simulink subsystem "sim_battery_subsystem"  (R2023a)
settings: Solver=VariableStepAuto  StartTime=0.0  StopTime=10.0  RelTol=1e-3
undefined symbols (not defined in the file or in its folder): battery_builder_rtmsupport, gcbh
libraries: nesl_utility x14, GD_Batterymodel_6_lib x8, fl_lib x7, BatteryCurrentManagement x1, batt_lib x1, BatteryBalancing x1, simulink x1, SimscapeFluids_lib x1
(part 2 of 2)

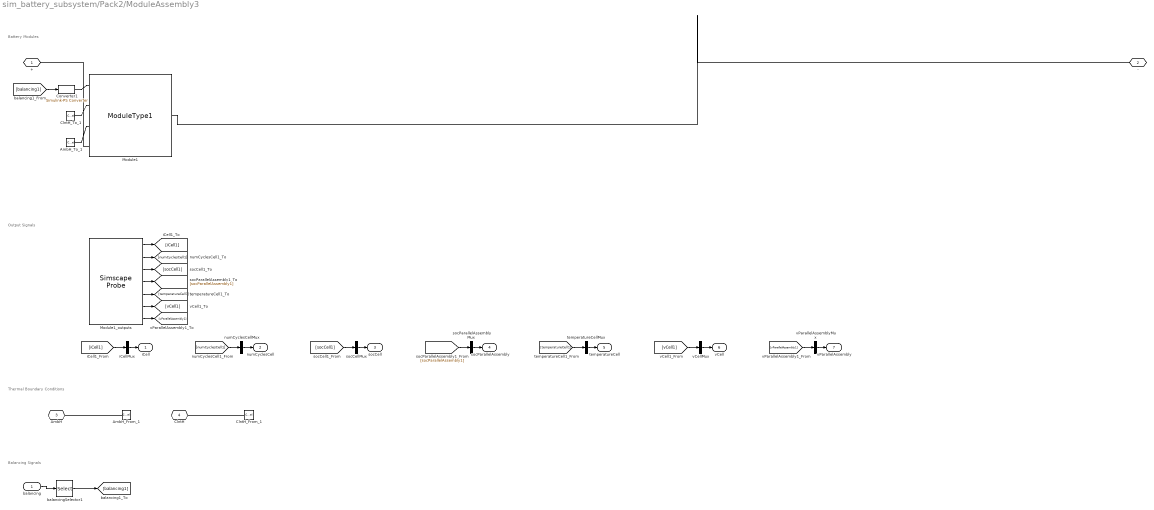
== system sim_battery_subsystem/Pack2/ModuleAssembly3 ==
  note: Balancing Signals
  note: Thermal Boundary Conditions
  note: Output Signals
  note: Battery Modules
  balancing : Inport  PortDimensions=14
  AmbH_From_1 : ConnectionLabel  Label=ambH_1
  AmbH_To_1 : ConnectionLabel  Label=ambH_1
  ClntH_From_1 : ConnectionLabel  Label=clntH_1
  ClntH_To_1 : ConnectionLabel  Label=clntH_1
  Converter1 : nesl_utility/Simulink-PS Converter  PhysicalDomain=network_engine_domain  SubClassName=ps_input  LeftPortType=input  RightPortType=output  PseudoPeriodic=off  Frequencies=[]  NoiseDistribution=none  NoiseParameters=[]  Unit=1  AffineConversion=off  FilteringAndDerivatives=provide  SimscapeFilterOrder=1  InputFilterTimeConstant=0.001  UdotUserProvided=0
  Module1 : GD_Batterymodel_6_lib/Modules/ModuleType1  SOC_vecCell=ModuleType1.SOC_vecCell  T_vecCell=ModuleType1.T_vecCell K  V0_matCell=ModuleType1.V0_matCell V  V_rangeCell=ModuleType1.V_rangeCell V  R0_matCell=ModuleType1.R0_matCell Ohm  AHCell=ModuleType1.AHCell A*hr  extrapolation_optionCell=simscape.enum.extrapolation.nearest  R1_matCell=ModuleType1.R1_matCell Ohm  tau1_matCell=ModuleType1.tau1_matCell s  R2_matCell=ModuleType1.R2_matCell Ohm  tau2_matCell=ModuleType1.tau2_matCell s  thermal_massCell=ModuleType1.thermal_massCell J/K  CoolantResistance=ModuleType1.CoolantResistance K/W  AmbientResistance=ModuleType1.AmbientResistance K/W  CellBalancingClosedResistance=ModuleType1.CellBalancingClosedResistance Ohm  CellBalancingOpenConductance=ModuleType1.CellBalancingOpenConductance 1/Ohm  CellBalancingThreshold=ModuleType1.CellBalancingThreshold  CellBalancingResistance=ModuleType1.CellBalancingResistance Ohm  P=3  S=14  iCell_specify=on  iCell_priority=None  iCell=ModuleAssembly3.Module1.iCell A  iCell_nominal_specify=off  iCell_nominal_unit=A  iCell_nominal_value=1  vCell_specify=on  vCell_priority=None  vCell=ModuleAssembly3.Module1.vCell V  vCell_nominal_specify=off  vCell_nominal_unit=V  vCell_nominal_value=1  socCell_specify=on  socCell_priority=High  socCell=ModuleAssembly3.Module1.socCell  socCell_nominal_specify=off  socCell_nominal_unit=1  socCell_nominal_value=1  numCyclesCell_specify=on  numCyclesCell_priority=High  numCyclesCell=ModuleAssembly3.Module1.numCyclesCell  numCyclesCell_nominal_specify=off  numCyclesCell_nominal_unit=1  numCyclesCell_nominal_value=1  temperatureCell_specify=on  temperatureCell_priority=High  temperatureCell=ModuleAssembly3.Module1.temperatureCell K  temperatureCell_nominal_specify=off  temperatureCell_nominal_unit=K  temperatureCell_nominal_value=1  vParallelAssembly_specify=on  vParallelAssembly_priority=None  vParallelAssembly=ModuleAssembly3.Module1.vParallelAssembly V  vParallelAssembly_nominal_specify=off  vParallelAssembly_nominal_unit=V  vParallelAssembly_nominal_value=1  socParallelAssembly_specify=on  socParallelAssembly_priority=None  socParallelAssembly=ModuleAssembly3.Module1.socParallelAssembly  socParallelAssembly_nominal_specify=off  socParallelAssembly_nominal_unit=1  socParallelAssembly_nominal_value=1
      settings: InternalSimscapePortConfiguration="{\"Bottom\":[{\"id\":\"n\",\"label\":\"-\",\"type\":\"foundation.electrical.electrical\"}],\"Left\":[{\"id\":\"enableCellBalancing\",\"label\":\"CB\",\"type\":\"input\"},{\"id\":\"ClntH\",\"label\":\"CH\",\"type\":\"foundation.thermal.thermal\"},{\"id\":\"AmbH\",\"label\":\"AH\",\"type\":\"foundation.thermal.thermal\"}],\"Right\":[],\"Top\":[{\"id\":\"p\",\"label\":\"+\",\"type\":\"foundation.electrical.electrical\"}]}"
  Module1_outputs : SimscapeProbe  BoundBlock=152  Variables={iCell, numCyclesCell, socCell, socParallelAssembly, temperatureCell, vCell, vParallelAssembly}
  balancingSelector1 : Selector  InputPortWidth=14  IndexOptions=Index vector (dialog)  Indices="[1   2   3   4   5   6   7   8   9  10  11  12  13  14]"  OutputSizes=1
  iCellMux : Mux  Inputs=1
  numCyclesCellMux : Mux  Inputs=1
  socCellMux : Mux  Inputs=1
  socParallelAssemblyMux : Mux  Inputs=1
  temperatureCellMux : Mux  Inputs=1
  vCellMux : Mux  Inputs=1
  vParallelAssemblyMux : Mux  Inputs=1
  + : PMIOPort  Side=Left
  - : PMIOPort  Port=2  Side=Right
  AmbH : PMIOPort  Port=3  Side=Right  ConnectionType=Connection: foundation.thermal.thermal
  ClntH : PMIOPort  Port=4  Side=Right  ConnectionType=Connection: foundation.thermal.thermal
  iCell : Outport
  numCyclesCell : Outport  Port=2
  socCell : Outport  Port=3
  socParallelAssembly : Outport  Port=4
  temperatureCell : Outport  Port=5
  vCell : Outport  Port=6
  vParallelAssembly : Outport  Port=7
  wires:
  balancingSelector1/1 -> [balancing1]
  balancing/1 -> balancingSelector1/1
  [balancing1] -> Converter1/1
  [vParallelAssembly1] -> vParallelAssemblyMux/1
  vParallelAssemblyMux/1 -> vParallelAssembly/1
  Module1_outputs/7 -> [vParallelAssembly1]
  [vCell1] -> vCellMux/1
  vCellMux/1 -> vCell/1
  Module1_outputs/6 -> [vCell1]
  [temperatureCell1] -> temperatureCellMux/1
  temperatureCellMux/1 -> temperatureCell/1
  Module1_outputs/5 -> [temperatureCell1]
  [socParallelAssembly1] -> socParallelAssemblyMux/1
  socParallelAssemblyMux/1 -> socParallelAssembly/1
  Module1_outputs/4 -> [socParallelAssembly1]
  [socCell1] -> socCellMux/1
  socCellMux/1 -> socCell/1
  Module1_outputs/3 -> [socCell1]
  [numCyclesCell1] -> numCyclesCellMux/1
  numCyclesCellMux/1 -> numCyclesCell/1
  Module1_outputs/2 -> [numCyclesCell1]
  [iCell1] -> iCellMux/1
  iCellMux/1 -> iCell/1
  Module1_outputs/1 -> [iCell1]
  connections:
  Converter1/RConn1 -- Module1/LConn1
  ClntH_From_1/LConn1 -- ClntH/RConn1
  ClntH_To_1/LConn1 -- Module1/LConn2
  AmbH_From_1/LConn1 -- AmbH/RConn1
  AmbH_To_1/LConn1 -- Module1/LConn3
  Module1/RConn1 -- -/RConn1
  Module1/LConn4 -- +/RConn1

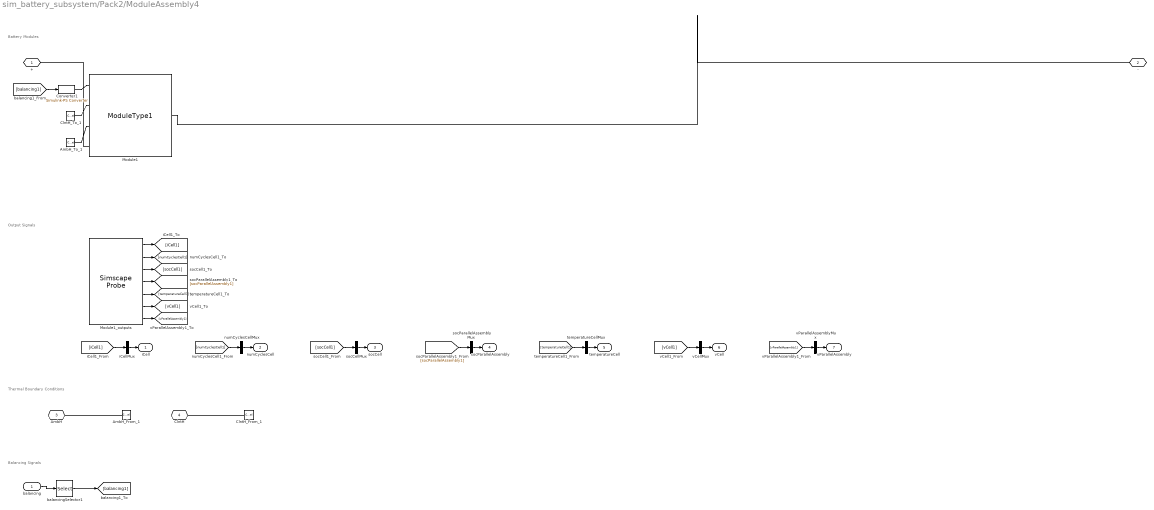
== system sim_battery_subsystem/Pack2/ModuleAssembly4 ==
  note: Balancing Signals
  note: Thermal Boundary Conditions
  note: Output Signals
  note: Battery Modules
  balancing : Inport  PortDimensions=14
  AmbH_From_1 : ConnectionLabel  Label=ambH_1
  AmbH_To_1 : ConnectionLabel  Label=ambH_1
  ClntH_From_1 : ConnectionLabel  Label=clntH_1
  ClntH_To_1 : ConnectionLabel  Label=clntH_1
  Converter1 : nesl_utility/Simulink-PS Converter  PhysicalDomain=network_engine_domain  SubClassName=ps_input  LeftPortType=input  RightPortType=output  PseudoPeriodic=off  Frequencies=[]  NoiseDistribution=none  NoiseParameters=[]  Unit=1  AffineConversion=off  FilteringAndDerivatives=provide  SimscapeFilterOrder=1  InputFilterTimeConstant=0.001  UdotUserProvided=0
  Module1 : GD_Batterymodel_6_lib/Modules/ModuleType1  SOC_vecCell=ModuleType1.SOC_vecCell  T_vecCell=ModuleType1.T_vecCell K  V0_matCell=ModuleType1.V0_matCell V  V_rangeCell=ModuleType1.V_rangeCell V  R0_matCell=ModuleType1.R0_matCell Ohm  AHCell=ModuleType1.AHCell A*hr  extrapolation_optionCell=simscape.enum.extrapolation.nearest  R1_matCell=ModuleType1.R1_matCell Ohm  tau1_matCell=ModuleType1.tau1_matCell s  R2_matCell=ModuleType1.R2_matCell Ohm  tau2_matCell=ModuleType1.tau2_matCell s  thermal_massCell=ModuleType1.thermal_massCell J/K  CoolantResistance=ModuleType1.CoolantResistance K/W  AmbientResistance=ModuleType1.AmbientResistance K/W  CellBalancingClosedResistance=ModuleType1.CellBalancingClosedResistance Ohm  CellBalancingOpenConductance=ModuleType1.CellBalancingOpenConductance 1/Ohm  CellBalancingThreshold=ModuleType1.CellBalancingThreshold  CellBalancingResistance=ModuleType1.CellBalancingResistance Ohm  P=3  S=14  iCell_specify=on  iCell_priority=None  iCell=ModuleAssembly4.Module1.iCell A  iCell_nominal_specify=off  iCell_nominal_unit=A  iCell_nominal_value=1  vCell_specify=on  vCell_priority=None  vCell=ModuleAssembly4.Module1.vCell V  vCell_nominal_specify=off  vCell_nominal_unit=V  vCell_nominal_value=1  socCell_specify=on  socCell_priority=High  socCell=ModuleAssembly4.Module1.socCell  socCell_nominal_specify=off  socCell_nominal_unit=1  socCell_nominal_value=1  numCyclesCell_specify=on  numCyclesCell_priority=High  numCyclesCell=ModuleAssembly4.Module1.numCyclesCell  numCyclesCell_nominal_specify=off  numCyclesCell_nominal_unit=1  numCyclesCell_nominal_value=1  temperatureCell_specify=on  temperatureCell_priority=High  temperatureCell=ModuleAssembly4.Module1.temperatureCell K  temperatureCell_nominal_specify=off  temperatureCell_nominal_unit=K  temperatureCell_nominal_value=1  vParallelAssembly_specify=on  vParallelAssembly_priority=None  vParallelAssembly=ModuleAssembly4.Module1.vParallelAssembly V  vParallelAssembly_nominal_specify=off  vParallelAssembly_nominal_unit=V  vParallelAssembly_nominal_value=1  socParallelAssembly_specify=on  socParallelAssembly_priority=None  socParallelAssembly=ModuleAssembly4.Module1.socParallelAssembly  socParallelAssembly_nominal_specify=off  socParallelAssembly_nominal_unit=1  socParallelAssembly_nominal_value=1
      settings: InternalSimscapePortConfiguration="{\"Bottom\":[{\"id\":\"n\",\"label\":\"-\",\"type\":\"foundation.electrical.electrical\"}],\"Left\":[{\"id\":\"enableCellBalancing\",\"label\":\"CB\",\"type\":\"input\"},{\"id\":\"ClntH\",\"label\":\"CH\",\"type\":\"foundation.thermal.thermal\"},{\"id\":\"AmbH\",\"label\":\"AH\",\"type\":\"foundation.thermal.thermal\"}],\"Right\":[],\"Top\":[{\"id\":\"p\",\"label\":\"+\",\"type\":\"foundation.electrical.electrical\"}]}"
  Module1_outputs : SimscapeProbe  BoundBlock=200  Variables={iCell, numCyclesCell, socCell, socParallelAssembly, temperatureCell, vCell, vParallelAssembly}
  balancingSelector1 : Selector  InputPortWidth=14  IndexOptions=Index vector (dialog)  Indices="[1   2   3   4   5   6   7   8   9  10  11  12  13  14]"  OutputSizes=1
  iCellMux : Mux  Inputs=1
  numCyclesCellMux : Mux  Inputs=1
  socCellMux : Mux  Inputs=1
  socParallelAssemblyMux : Mux  Inputs=1
  temperatureCellMux : Mux  Inputs=1
  vCellMux : Mux  Inputs=1
  vParallelAssemblyMux : Mux  Inputs=1
  + : PMIOPort  Side=Left
  - : PMIOPort  Port=2  Side=Right
  AmbH : PMIOPort  Port=3  Side=Right  ConnectionType=Connection: foundation.thermal.thermal
  ClntH : PMIOPort  Port=4  Side=Right  ConnectionType=Connection: foundation.thermal.thermal
  iCell : Outport
  numCyclesCell : Outport  Port=2
  socCell : Outport  Port=3
  socParallelAssembly : Outport  Port=4
  temperatureCell : Outport  Port=5
  vCell : Outport  Port=6
  vParallelAssembly : Outport  Port=7
  wires:
  balancingSelector1/1 -> [balancing1]
  balancing/1 -> balancingSelector1/1
  [balancing1] -> Converter1/1
  [vParallelAssembly1] -> vParallelAssemblyMux/1
  vParallelAssemblyMux/1 -> vParallelAssembly/1
  Module1_outputs/7 -> [vParallelAssembly1]
  [vCell1] -> vCellMux/1
  vCellMux/1 -> vCell/1
  Module1_outputs/6 -> [vCell1]
  [temperatureCell1] -> temperatureCellMux/1
  temperatureCellMux/1 -> temperatureCell/1
  Module1_outputs/5 -> [temperatureCell1]
  [socParallelAssembly1] -> socParallelAssemblyMux/1
  socParallelAssemblyMux/1 -> socParallelAssembly/1
  Module1_outputs/4 -> [socParallelAssembly1]
  [socCell1] -> socCellMux/1
  socCellMux/1 -> socCell/1
  Module1_outputs/3 -> [socCell1]
  [numCyclesCell1] -> numCyclesCellMux/1
  numCyclesCellMux/1 -> numCyclesCell/1
  Module1_outputs/2 -> [numCyclesCell1]
  [iCell1] -> iCellMux/1
  iCellMux/1 -> iCell/1
  Module1_outputs/1 -> [iCell1]
  connections:
  Converter1/RConn1 -- Module1/LConn1
  ClntH_From_1/LConn1 -- ClntH/RConn1
  ClntH_To_1/LConn1 -- Module1/LConn2
  AmbH_From_1/LConn1 -- AmbH/RConn1
  AmbH_To_1/LConn1 -- Module1/LConn3
  Module1/RConn1 -- -/RConn1
  Module1/LConn4 -- +/RConn1

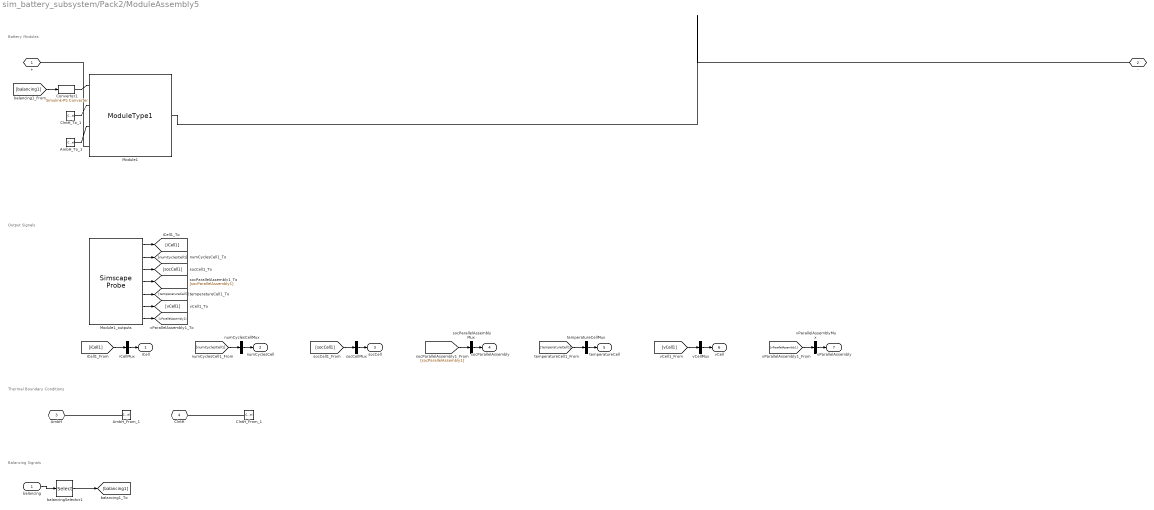
== system sim_battery_subsystem/Pack2/ModuleAssembly5 ==
  note: Balancing Signals
  note: Thermal Boundary Conditions
  note: Output Signals
  note: Battery Modules
  balancing : Inport  PortDimensions=14
  AmbH_From_1 : ConnectionLabel  Label=ambH_1
  AmbH_To_1 : ConnectionLabel  Label=ambH_1
  ClntH_From_1 : ConnectionLabel  Label=clntH_1
  ClntH_To_1 : ConnectionLabel  Label=clntH_1
  Converter1 : nesl_utility/Simulink-PS Converter  PhysicalDomain=network_engine_domain  SubClassName=ps_input  LeftPortType=input  RightPortType=output  PseudoPeriodic=off  Frequencies=[]  NoiseDistribution=none  NoiseParameters=[]  Unit=1  AffineConversion=off  FilteringAndDerivatives=provide  SimscapeFilterOrder=1  InputFilterTimeConstant=0.001  UdotUserProvided=0
  Module1 : GD_Batterymodel_6_lib/Modules/ModuleType1  SOC_vecCell=ModuleType1.SOC_vecCell  T_vecCell=ModuleType1.T_vecCell K  V0_matCell=ModuleType1.V0_matCell V  V_rangeCell=ModuleType1.V_rangeCell V  R0_matCell=ModuleType1.R0_matCell Ohm  AHCell=ModuleType1.AHCell A*hr  extrapolation_optionCell=simscape.enum.extrapolation.nearest  R1_matCell=ModuleType1.R1_matCell Ohm  tau1_matCell=ModuleType1.tau1_matCell s  R2_matCell=ModuleType1.R2_matCell Ohm  tau2_matCell=ModuleType1.tau2_matCell s  thermal_massCell=ModuleType1.thermal_massCell J/K  CoolantResistance=ModuleType1.CoolantResistance K/W  AmbientResistance=ModuleType1.AmbientResistance K/W  CellBalancingClosedResistance=ModuleType1.CellBalancingClosedResistance Ohm  CellBalancingOpenConductance=ModuleType1.CellBalancingOpenConductance 1/Ohm  CellBalancingThreshold=ModuleType1.CellBalancingThreshold  CellBalancingResistance=ModuleType1.CellBalancingResistance Ohm  P=3  S=14  iCell_specify=on  iCell_priority=None  iCell=ModuleAssembly5.Module1.iCell A  iCell_nominal_specify=off  iCell_nominal_unit=A  iCell_nominal_value=1  vCell_specify=on  vCell_priority=None  vCell=ModuleAssembly5.Module1.vCell V  vCell_nominal_specify=off  vCell_nominal_unit=V  vCell_nominal_value=1  socCell_specify=on  socCell_priority=High  socCell=ModuleAssembly5.Module1.socCell  socCell_nominal_specify=off  socCell_nominal_unit=1  socCell_nominal_value=1  numCyclesCell_specify=on  numCyclesCell_priority=High  numCyclesCell=ModuleAssembly5.Module1.numCyclesCell  numCyclesCell_nominal_specify=off  numCyclesCell_nominal_unit=1  numCyclesCell_nominal_value=1  temperatureCell_specify=on  temperatureCell_priority=High  temperatureCell=ModuleAssembly5.Module1.temperatureCell K  temperatureCell_nominal_specify=off  temperatureCell_nominal_unit=K  temperatureCell_nominal_value=1  vParallelAssembly_specify=on  vParallelAssembly_priority=None  vParallelAssembly=ModuleAssembly5.Module1.vParallelAssembly V  vParallelAssembly_nominal_specify=off  vParallelAssembly_nominal_unit=V  vParallelAssembly_nominal_value=1  socParallelAssembly_specify=on  socParallelAssembly_priority=None  socParallelAssembly=ModuleAssembly5.Module1.socParallelAssembly  socParallelAssembly_nominal_specify=off  socParallelAssembly_nominal_unit=1  socParallelAssembly_nominal_value=1
      settings: InternalSimscapePortConfiguration="{\"Bottom\":[{\"id\":\"n\",\"label\":\"-\",\"type\":\"foundation.electrical.electrical\"}],\"Left\":[{\"id\":\"enableCellBalancing\",\"label\":\"CB\",\"type\":\"input\"},{\"id\":\"ClntH\",\"label\":\"CH\",\"type\":\"foundation.thermal.thermal\"},{\"id\":\"AmbH\",\"label\":\"AH\",\"type\":\"foundation.thermal.thermal\"}],\"Right\":[],\"Top\":[{\"id\":\"p\",\"label\":\"+\",\"type\":\"foundation.electrical.electrical\"}]}"
  Module1_outputs : SimscapeProbe  BoundBlock=248  Variables={iCell, numCyclesCell, socCell, socParallelAssembly, temperatureCell, vCell, vParallelAssembly}
  balancingSelector1 : Selector  InputPortWidth=14  IndexOptions=Index vector (dialog)  Indices="[1   2   3   4   5   6   7   8   9  10  11  12  13  14]"  OutputSizes=1
  iCellMux : Mux  Inputs=1
  numCyclesCellMux : Mux  Inputs=1
  socCellMux : Mux  Inputs=1
  socParallelAssemblyMux : Mux  Inputs=1
  temperatureCellMux : Mux  Inputs=1
  vCellMux : Mux  Inputs=1
  vParallelAssemblyMux : Mux  Inputs=1
  + : PMIOPort  Side=Left
  - : PMIOPort  Port=2  Side=Right
  AmbH : PMIOPort  Port=3  Side=Right  ConnectionType=Connection: foundation.thermal.thermal
  ClntH : PMIOPort  Port=4  Side=Right  ConnectionType=Connection: foundation.thermal.thermal
  iCell : Outport
  numCyclesCell : Outport  Port=2
  socCell : Outport  Port=3
  socParallelAssembly : Outport  Port=4
  temperatureCell : Outport  Port=5
  vCell : Outport  Port=6
  vParallelAssembly : Outport  Port=7
  wires:
  balancingSelector1/1 -> [balancing1]
  balancing/1 -> balancingSelector1/1
  [balancing1] -> Converter1/1
  [vParallelAssembly1] -> vParallelAssemblyMux/1
  vParallelAssemblyMux/1 -> vParallelAssembly/1
  Module1_outputs/7 -> [vParallelAssembly1]
  [vCell1] -> vCellMux/1
  vCellMux/1 -> vCell/1
  Module1_outputs/6 -> [vCell1]
  [temperatureCell1] -> temperatureCellMux/1
  temperatureCellMux/1 -> temperatureCell/1
  Module1_outputs/5 -> [temperatureCell1]
  [socParallelAssembly1] -> socParallelAssemblyMux/1
  socParallelAssemblyMux/1 -> socParallelAssembly/1
  Module1_outputs/4 -> [socParallelAssembly1]
  [socCell1] -> socCellMux/1
  socCellMux/1 -> socCell/1
  Module1_outputs/3 -> [socCell1]
  [numCyclesCell1] -> numCyclesCellMux/1
  numCyclesCellMux/1 -> numCyclesCell/1
  Module1_outputs/2 -> [numCyclesCell1]
  [iCell1] -> iCellMux/1
  iCellMux/1 -> iCell/1
  Module1_outputs/1 -> [iCell1]
  connections:
  Converter1/RConn1 -- Module1/LConn1
  ClntH_From_1/LConn1 -- ClntH/RConn1
  ClntH_To_1/LConn1 -- Module1/LConn2
  AmbH_From_1/LConn1 -- AmbH/RConn1
  AmbH_To_1/LConn1 -- Module1/LConn3
  Module1/RConn1 -- -/RConn1
  Module1/LConn4 -- +/RConn1

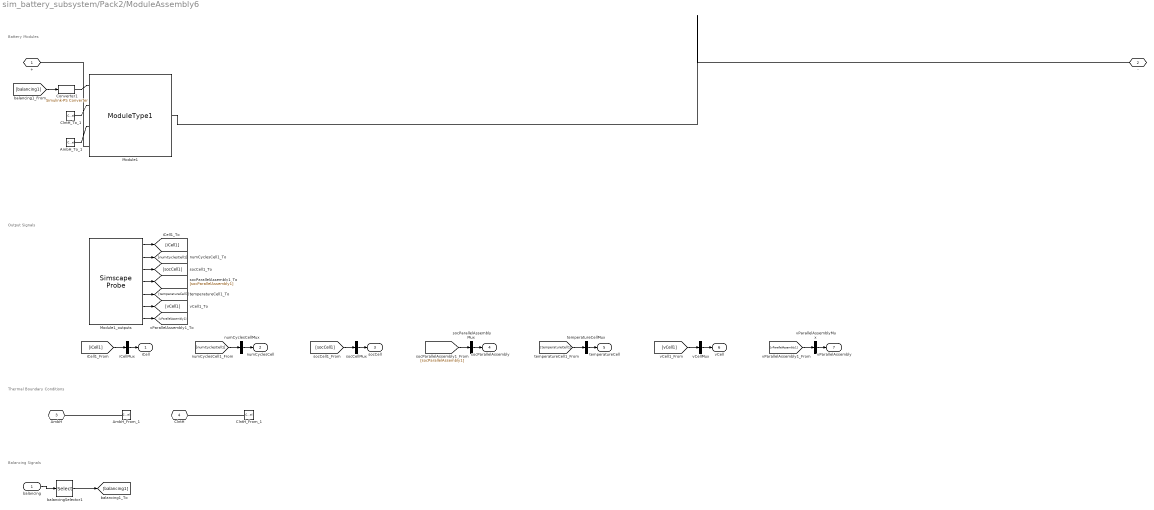
== system sim_battery_subsystem/Pack2/ModuleAssembly6 ==
  note: Balancing Signals
  note: Thermal Boundary Conditions
  note: Output Signals
  note: Battery Modules
  balancing : Inport  PortDimensions=14
  AmbH_From_1 : ConnectionLabel  Label=ambH_1
  AmbH_To_1 : ConnectionLabel  Label=ambH_1
  ClntH_From_1 : ConnectionLabel  Label=clntH_1
  ClntH_To_1 : ConnectionLabel  Label=clntH_1
  Converter1 : nesl_utility/Simulink-PS Converter  PhysicalDomain=network_engine_domain  SubClassName=ps_input  LeftPortType=input  RightPortType=output  PseudoPeriodic=off  Frequencies=[]  NoiseDistribution=none  NoiseParameters=[]  Unit=1  AffineConversion=off  FilteringAndDerivatives=provide  SimscapeFilterOrder=1  InputFilterTimeConstant=0.001  UdotUserProvided=0
  Module1 : GD_Batterymodel_6_lib/Modules/ModuleType1  SOC_vecCell=ModuleType1.SOC_vecCell  T_vecCell=ModuleType1.T_vecCell K  V0_matCell=ModuleType1.V0_matCell V  V_rangeCell=ModuleType1.V_rangeCell V  R0_matCell=ModuleType1.R0_matCell Ohm  AHCell=ModuleType1.AHCell A*hr  extrapolation_optionCell=simscape.enum.extrapolation.nearest  R1_matCell=ModuleType1.R1_matCell Ohm  tau1_matCell=ModuleType1.tau1_matCell s  R2_matCell=ModuleType1.R2_matCell Ohm  tau2_matCell=ModuleType1.tau2_matCell s  thermal_massCell=ModuleType1.thermal_massCell J/K  CoolantResistance=ModuleType1.CoolantResistance K/W  AmbientResistance=ModuleType1.AmbientResistance K/W  CellBalancingClosedResistance=ModuleType1.CellBalancingClosedResistance Ohm  CellBalancingOpenConductance=ModuleType1.CellBalancingOpenConductance 1/Ohm  CellBalancingThreshold=ModuleType1.CellBalancingThreshold  CellBalancingResistance=ModuleType1.CellBalancingResistance Ohm  P=3  S=14  iCell_specify=on  iCell_priority=None  iCell=ModuleAssembly6.Module1.iCell A  iCell_nominal_specify=off  iCell_nominal_unit=A  iCell_nominal_value=1  vCell_specify=on  vCell_priority=None  vCell=ModuleAssembly6.Module1.vCell V  vCell_nominal_specify=off  vCell_nominal_unit=V  vCell_nominal_value=1  socCell_specify=on  socCell_priority=High  socCell=ModuleAssembly6.Module1.socCell  socCell_nominal_specify=off  socCell_nominal_unit=1  socCell_nominal_value=1  numCyclesCell_specify=on  numCyclesCell_priority=High  numCyclesCell=ModuleAssembly6.Module1.numCyclesCell  numCyclesCell_nominal_specify=off  numCyclesCell_nominal_unit=1  numCyclesCell_nominal_value=1  temperatureCell_specify=on  temperatureCell_priority=High  temperatureCell=ModuleAssembly6.Module1.temperatureCell K  temperatureCell_nominal_specify=off  temperatureCell_nominal_unit=K  temperatureCell_nominal_value=1  vParallelAssembly_specify=on  vParallelAssembly_priority=None  vParallelAssembly=ModuleAssembly6.Module1.vParallelAssembly V  vParallelAssembly_nominal_specify=off  vParallelAssembly_nominal_unit=V  vParallelAssembly_nominal_value=1  socParallelAssembly_specify=on  socParallelAssembly_priority=None  socParallelAssembly=ModuleAssembly6.Module1.socParallelAssembly  socParallelAssembly_nominal_specify=off  socParallelAssembly_nominal_unit=1  socParallelAssembly_nominal_value=1
      settings: InternalSimscapePortConfiguration="{\"Bottom\":[{\"id\":\"n\",\"label\":\"-\",\"type\":\"foundation.electrical.electrical\"}],\"Left\":[{\"id\":\"enableCellBalancing\",\"label\":\"CB\",\"type\":\"input\"},{\"id\":\"ClntH\",\"label\":\"CH\",\"type\":\"foundation.thermal.thermal\"},{\"id\":\"AmbH\",\"label\":\"AH\",\"type\":\"foundation.thermal.thermal\"}],\"Right\":[],\"Top\":[{\"id\":\"p\",\"label\":\"+\",\"type\":\"foundation.electrical.electrical\"}]}"
  Module1_outputs : SimscapeProbe  BoundBlock=296  Variables={iCell, numCyclesCell, socCell, socParallelAssembly, temperatureCell, vCell, vParallelAssembly}
  balancingSelector1 : Selector  InputPortWidth=14  IndexOptions=Index vector (dialog)  Indices="[1   2   3   4   5   6   7   8   9  10  11  12  13  14]"  OutputSizes=1
  iCellMux : Mux  Inputs=1
  numCyclesCellMux : Mux  Inputs=1
  socCellMux : Mux  Inputs=1
  socParallelAssemblyMux : Mux  Inputs=1
  temperatureCellMux : Mux  Inputs=1
  vCellMux : Mux  Inputs=1
  vParallelAssemblyMux : Mux  Inputs=1
  + : PMIOPort  Side=Left
  - : PMIOPort  Port=2  Side=Right
  AmbH : PMIOPort  Port=3  Side=Right  ConnectionType=Connection: foundation.thermal.thermal
  ClntH : PMIOPort  Port=4  Side=Right  ConnectionType=Connection: foundation.thermal.thermal
  iCell : Outport
  numCyclesCell : Outport  Port=2
  socCell : Outport  Port=3
  socParallelAssembly : Outport  Port=4
  temperatureCell : Outport  Port=5
  vCell : Outport  Port=6
  vParallelAssembly : Outport  Port=7
  wires:
  balancingSelector1/1 -> [balancing1]
  balancing/1 -> balancingSelector1/1
  [balancing1] -> Converter1/1
  [vParallelAssembly1] -> vParallelAssemblyMux/1
  vParallelAssemblyMux/1 -> vParallelAssembly/1
  Module1_outputs/7 -> [vParallelAssembly1]
  [vCell1] -> vCellMux/1
  vCellMux/1 -> vCell/1
  Module1_outputs/6 -> [vCell1]
  [temperatureCell1] -> temperatureCellMux/1
  temperatureCellMux/1 -> temperatureCell/1
  Module1_outputs/5 -> [temperatureCell1]
  [socParallelAssembly1] -> socParallelAssemblyMux/1
  socParallelAssemblyMux/1 -> socParallelAssembly/1
  Module1_outputs/4 -> [socParallelAssembly1]
  [socCell1] -> socCellMux/1
  socCellMux/1 -> socCell/1
  Module1_outputs/3 -> [socCell1]
  [numCyclesCell1] -> numCyclesCellMux/1
  numCyclesCellMux/1 -> numCyclesCell/1
  Module1_outputs/2 -> [numCyclesCell1]
  [iCell1] -> iCellMux/1
  iCellMux/1 -> iCell/1
  Module1_outputs/1 -> [iCell1]
  connections:
  Converter1/RConn1 -- Module1/LConn1
  ClntH_From_1/LConn1 -- ClntH/RConn1
  ClntH_To_1/LConn1 -- Module1/LConn2
  AmbH_From_1/LConn1 -- AmbH/RConn1
  AmbH_To_1/LConn1 -- Module1/LConn3
  Module1/RConn1 -- -/RConn1
  Module1/LConn4 -- +/RConn1

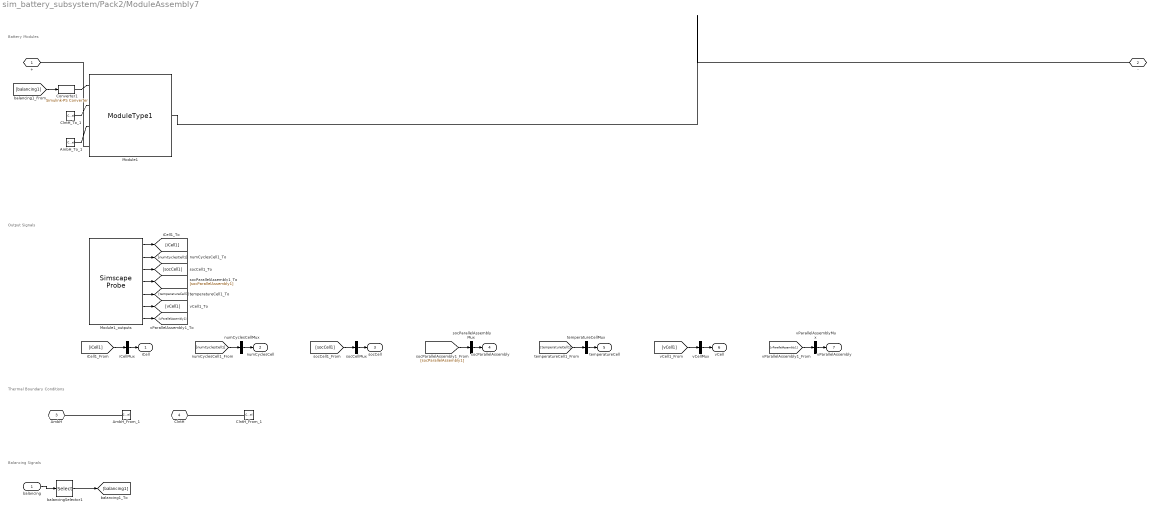
== system sim_battery_subsystem/Pack2/ModuleAssembly7 ==
  note: Balancing Signals
  note: Thermal Boundary Conditions
  note: Output Signals
  note: Battery Modules
  balancing : Inport  PortDimensions=14
  AmbH_From_1 : ConnectionLabel  Label=ambH_1
  AmbH_To_1 : ConnectionLabel  Label=ambH_1
  ClntH_From_1 : ConnectionLabel  Label=clntH_1
  ClntH_To_1 : ConnectionLabel  Label=clntH_1
  Converter1 : nesl_utility/Simulink-PS Converter  PhysicalDomain=network_engine_domain  SubClassName=ps_input  LeftPortType=input  RightPortType=output  PseudoPeriodic=off  Frequencies=[]  NoiseDistribution=none  NoiseParameters=[]  Unit=1  AffineConversion=off  FilteringAndDerivatives=provide  SimscapeFilterOrder=1  InputFilterTimeConstant=0.001  UdotUserProvided=0
  Module1 : GD_Batterymodel_6_lib/Modules/ModuleType1  SOC_vecCell=ModuleType1.SOC_vecCell  T_vecCell=ModuleType1.T_vecCell K  V0_matCell=ModuleType1.V0_matCell V  V_rangeCell=ModuleType1.V_rangeCell V  R0_matCell=ModuleType1.R0_matCell Ohm  AHCell=ModuleType1.AHCell A*hr  extrapolation_optionCell=simscape.enum.extrapolation.nearest  R1_matCell=ModuleType1.R1_matCell Ohm  tau1_matCell=ModuleType1.tau1_matCell s  R2_matCell=ModuleType1.R2_matCell Ohm  tau2_matCell=ModuleType1.tau2_matCell s  thermal_massCell=ModuleType1.thermal_massCell J/K  CoolantResistance=ModuleType1.CoolantResistance K/W  AmbientResistance=ModuleType1.AmbientResistance K/W  CellBalancingClosedResistance=ModuleType1.CellBalancingClosedResistance Ohm  CellBalancingOpenConductance=ModuleType1.CellBalancingOpenConductance 1/Ohm  CellBalancingThreshold=ModuleType1.CellBalancingThreshold  CellBalancingResistance=ModuleType1.CellBalancingResistance Ohm  P=3  S=14  iCell_specify=on  iCell_priority=None  iCell=ModuleAssembly7.Module1.iCell A  iCell_nominal_specify=off  iCell_nominal_unit=A  iCell_nominal_value=1  vCell_specify=on  vCell_priority=None  vCell=ModuleAssembly7.Module1.vCell V  vCell_nominal_specify=off  vCell_nominal_unit=V  vCell_nominal_value=1  socCell_specify=on  socCell_priority=High  socCell=ModuleAssembly7.Module1.socCell  socCell_nominal_specify=off  socCell_nominal_unit=1  socCell_nominal_value=1  numCyclesCell_specify=on  numCyclesCell_priority=High  numCyclesCell=ModuleAssembly7.Module1.numCyclesCell  numCyclesCell_nominal_specify=off  numCyclesCell_nominal_unit=1  numCyclesCell_nominal_value=1  temperatureCell_specify=on  temperatureCell_priority=High  temperatureCell=ModuleAssembly7.Module1.temperatureCell K  temperatureCell_nominal_specify=off  temperatureCell_nominal_unit=K  temperatureCell_nominal_value=1  vParallelAssembly_specify=on  vParallelAssembly_priority=None  vParallelAssembly=ModuleAssembly7.Module1.vParallelAssembly V  vParallelAssembly_nominal_specify=off  vParallelAssembly_nominal_unit=V  vParallelAssembly_nominal_value=1  socParallelAssembly_specify=on  socParallelAssembly_priority=None  socParallelAssembly=ModuleAssembly7.Module1.socParallelAssembly  socParallelAssembly_nominal_specify=off  socParallelAssembly_nominal_unit=1  socParallelAssembly_nominal_value=1
      settings: InternalSimscapePortConfiguration="{\"Bottom\":[{\"id\":\"n\",\"label\":\"-\",\"type\":\"foundation.electrical.electrical\"}],\"Left\":[{\"id\":\"enableCellBalancing\",\"label\":\"CB\",\"type\":\"input\"},{\"id\":\"ClntH\",\"label\":\"CH\",\"type\":\"foundation.thermal.thermal\"},{\"id\":\"AmbH\",\"label\":\"AH\",\"type\":\"foundation.thermal.thermal\"}],\"Right\":[],\"Top\":[{\"id\":\"p\",\"label\":\"+\",\"type\":\"foundation.electrical.electrical\"}]}"
  Module1_outputs : SimscapeProbe  BoundBlock=344  Variables={iCell, numCyclesCell, socCell, socParallelAssembly, temperatureCell, vCell, vParallelAssembly}
  balancingSelector1 : Selector  InputPortWidth=14  IndexOptions=Index vector (dialog)  Indices="[1   2   3   4   5   6   7   8   9  10  11  12  13  14]"  OutputSizes=1
  iCellMux : Mux  Inputs=1
  numCyclesCellMux : Mux  Inputs=1
  socCellMux : Mux  Inputs=1
  socParallelAssemblyMux : Mux  Inputs=1
  temperatureCellMux : Mux  Inputs=1
  vCellMux : Mux  Inputs=1
  vParallelAssemblyMux : Mux  Inputs=1
  + : PMIOPort  Side=Left
  - : PMIOPort  Port=2  Side=Right
  AmbH : PMIOPort  Port=3  Side=Right  ConnectionType=Connection: foundation.thermal.thermal
  ClntH : PMIOPort  Port=4  Side=Right  ConnectionType=Connection: foundation.thermal.thermal
  iCell : Outport
  numCyclesCell : Outport  Port=2
  socCell : Outport  Port=3
  socParallelAssembly : Outport  Port=4
  temperatureCell : Outport  Port=5
  vCell : Outport  Port=6
  vParallelAssembly : Outport  Port=7
  wires:
  balancingSelector1/1 -> [balancing1]
  balancing/1 -> balancingSelector1/1
  [balancing1] -> Converter1/1
  [vParallelAssembly1] -> vParallelAssemblyMux/1
  vParallelAssemblyMux/1 -> vParallelAssembly/1
  Module1_outputs/7 -> [vParallelAssembly1]
  [vCell1] -> vCellMux/1
  vCellMux/1 -> vCell/1
  Module1_outputs/6 -> [vCell1]
  [temperatureCell1] -> temperatureCellMux/1
  temperatureCellMux/1 -> temperatureCell/1
  Module1_outputs/5 -> [temperatureCell1]
  [socParallelAssembly1] -> socParallelAssemblyMux/1
  socParallelAssemblyMux/1 -> socParallelAssembly/1
  Module1_outputs/4 -> [socParallelAssembly1]
  [socCell1] -> socCellMux/1
  socCellMux/1 -> socCell/1
  Module1_outputs/3 -> [socCell1]
  [numCyclesCell1] -> numCyclesCellMux/1
  numCyclesCellMux/1 -> numCyclesCell/1
  Module1_outputs/2 -> [numCyclesCell1]
  [iCell1] -> iCellMux/1
  iCellMux/1 -> iCell/1
  Module1_outputs/1 -> [iCell1]
  connections:
  Converter1/RConn1 -- Module1/LConn1
  ClntH_From_1/LConn1 -- ClntH/RConn1
  ClntH_To_1/LConn1 -- Module1/LConn2
  AmbH_From_1/LConn1 -- AmbH/RConn1
  AmbH_To_1/LConn1 -- Module1/LConn3
  Module1/RConn1 -- -/RConn1
  Module1/LConn4 -- +/RConn1

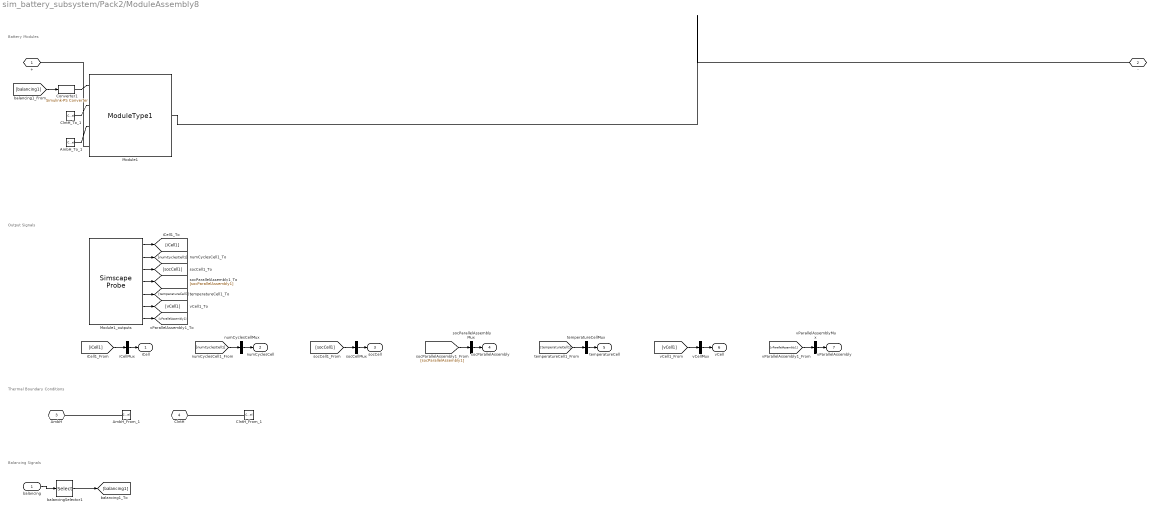
== system sim_battery_subsystem/Pack2/ModuleAssembly8 ==
  note: Balancing Signals
  note: Thermal Boundary Conditions
  note: Output Signals
  note: Battery Modules
  balancing : Inport  PortDimensions=14
  AmbH_From_1 : ConnectionLabel  Label=ambH_1
  AmbH_To_1 : ConnectionLabel  Label=ambH_1
  ClntH_From_1 : ConnectionLabel  Label=clntH_1
  ClntH_To_1 : ConnectionLabel  Label=clntH_1
  Converter1 : nesl_utility/Simulink-PS Converter  PhysicalDomain=network_engine_domain  SubClassName=ps_input  LeftPortType=input  RightPortType=output  PseudoPeriodic=off  Frequencies=[]  NoiseDistribution=none  NoiseParameters=[]  Unit=1  AffineConversion=off  FilteringAndDerivatives=provide  SimscapeFilterOrder=1  InputFilterTimeConstant=0.001  UdotUserProvided=0
  Module1 : GD_Batterymodel_6_lib/Modules/ModuleType1  SOC_vecCell=ModuleType1.SOC_vecCell  T_vecCell=ModuleType1.T_vecCell K  V0_matCell=ModuleType1.V0_matCell V  V_rangeCell=ModuleType1.V_rangeCell V  R0_matCell=ModuleType1.R0_matCell Ohm  AHCell=ModuleType1.AHCell A*hr  extrapolation_optionCell=simscape.enum.extrapolation.nearest  R1_matCell=ModuleType1.R1_matCell Ohm  tau1_matCell=ModuleType1.tau1_matCell s  R2_matCell=ModuleType1.R2_matCell Ohm  tau2_matCell=ModuleType1.tau2_matCell s  thermal_massCell=ModuleType1.thermal_massCell J/K  CoolantResistance=ModuleType1.CoolantResistance K/W  AmbientResistance=ModuleType1.AmbientResistance K/W  CellBalancingClosedResistance=ModuleType1.CellBalancingClosedResistance Ohm  CellBalancingOpenConductance=ModuleType1.CellBalancingOpenConductance 1/Ohm  CellBalancingThreshold=ModuleType1.CellBalancingThreshold  CellBalancingResistance=ModuleType1.CellBalancingResistance Ohm  P=3  S=14  iCell_specify=on  iCell_priority=None  iCell=ModuleAssembly8.Module1.iCell A  iCell_nominal_specify=off  iCell_nominal_unit=A  iCell_nominal_value=1  vCell_specify=on  vCell_priority=None  vCell=ModuleAssembly8.Module1.vCell V  vCell_nominal_specify=off  vCell_nominal_unit=V  vCell_nominal_value=1  socCell_specify=on  socCell_priority=High  socCell=ModuleAssembly8.Module1.socCell  socCell_nominal_specify=off  socCell_nominal_unit=1  socCell_nominal_value=1  numCyclesCell_specify=on  numCyclesCell_priority=High  numCyclesCell=ModuleAssembly8.Module1.numCyclesCell  numCyclesCell_nominal_specify=off  numCyclesCell_nominal_unit=1  numCyclesCell_nominal_value=1  temperatureCell_specify=on  temperatureCell_priority=High  temperatureCell=ModuleAssembly8.Module1.temperatureCell K  temperatureCell_nominal_specify=off  temperatureCell_nominal_unit=K  temperatureCell_nominal_value=1  vParallelAssembly_specify=on  vParallelAssembly_priority=None  vParallelAssembly=ModuleAssembly8.Module1.vParallelAssembly V  vParallelAssembly_nominal_specify=off  vParallelAssembly_nominal_unit=V  vParallelAssembly_nominal_value=1  socParallelAssembly_specify=on  socParallelAssembly_priority=None  socParallelAssembly=ModuleAssembly8.Module1.socParallelAssembly  socParallelAssembly_nominal_specify=off  socParallelAssembly_nominal_unit=1  socParallelAssembly_nominal_value=1
      settings: InternalSimscapePortConfiguration="{\"Bottom\":[{\"id\":\"n\",\"label\":\"-\",\"type\":\"foundation.electrical.electrical\"}],\"Left\":[{\"id\":\"enableCellBalancing\",\"label\":\"CB\",\"type\":\"input\"},{\"id\":\"ClntH\",\"label\":\"CH\",\"type\":\"foundation.thermal.thermal\"},{\"id\":\"AmbH\",\"label\":\"AH\",\"type\":\"foundation.thermal.thermal\"}],\"Right\":[],\"Top\":[{\"id\":\"p\",\"label\":\"+\",\"type\":\"foundation.electrical.electrical\"}]}"
  Module1_outputs : SimscapeProbe  BoundBlock=392  Variables={iCell, numCyclesCell, socCell, socParallelAssembly, temperatureCell, vCell, vParallelAssembly}
  balancingSelector1 : Selector  InputPortWidth=14  IndexOptions=Index vector (dialog)  Indices="[1   2   3   4   5   6   7   8   9  10  11  12  13  14]"  OutputSizes=1
  iCellMux : Mux  Inputs=1
  numCyclesCellMux : Mux  Inputs=1
  socCellMux : Mux  Inputs=1
  socParallelAssemblyMux : Mux  Inputs=1
  temperatureCellMux : Mux  Inputs=1
  vCellMux : Mux  Inputs=1
  vParallelAssemblyMux : Mux  Inputs=1
  + : PMIOPort  Side=Left
  - : PMIOPort  Port=2  Side=Right
  AmbH : PMIOPort  Port=3  Side=Right  ConnectionType=Connection: foundation.thermal.thermal
  ClntH : PMIOPort  Port=4  Side=Right  ConnectionType=Connection: foundation.thermal.thermal
  iCell : Outport
  numCyclesCell : Outport  Port=2
  socCell : Outport  Port=3
  socParallelAssembly : Outport  Port=4
  temperatureCell : Outport  Port=5
  vCell : Outport  Port=6
  vParallelAssembly : Outport  Port=7
  wires:
  balancingSelector1/1 -> [balancing1]
  balancing/1 -> balancingSelector1/1
  [balancing1] -> Converter1/1
  [vParallelAssembly1] -> vParallelAssemblyMux/1
  vParallelAssemblyMux/1 -> vParallelAssembly/1
  Module1_outputs/7 -> [vParallelAssembly1]
  [vCell1] -> vCellMux/1
  vCellMux/1 -> vCell/1
  Module1_outputs/6 -> [vCell1]
  [temperatureCell1] -> temperatureCellMux/1
  temperatureCellMux/1 -> temperatureCell/1
  Module1_outputs/5 -> [temperatureCell1]
  [socParallelAssembly1] -> socParallelAssemblyMux/1
  socParallelAssemblyMux/1 -> socParallelAssembly/1
  Module1_outputs/4 -> [socParallelAssembly1]
  [socCell1] -> socCellMux/1
  socCellMux/1 -> socCell/1
  Module1_outputs/3 -> [socCell1]
  [numCyclesCell1] -> numCyclesCellMux/1
  numCyclesCellMux/1 -> numCyclesCell/1
  Module1_outputs/2 -> [numCyclesCell1]
  [iCell1] -> iCellMux/1
  iCellMux/1 -> iCell/1
  Module1_outputs/1 -> [iCell1]
  connections:
  Converter1/RConn1 -- Module1/LConn1
  ClntH_From_1/LConn1 -- ClntH/RConn1
  ClntH_To_1/LConn1 -- Module1/LConn2
  AmbH_From_1/LConn1 -- AmbH/RConn1
  AmbH_To_1/LConn1 -- Module1/LConn3
  Module1/RConn1 -- -/RConn1
  Module1/LConn4 -- +/RConn1
